simulink model "addFM"  (R2024a)
settings: configuration reference "standardSILConfiguraitonParams" (kept outside this file)
libraries: simulink x2
settings Model: Creator=GTAR  LastModifiedBy=jerem
settings ConfigSetRef: SourceName=standardSILConfiguraitonParams  SourceLocation=Base Workspace

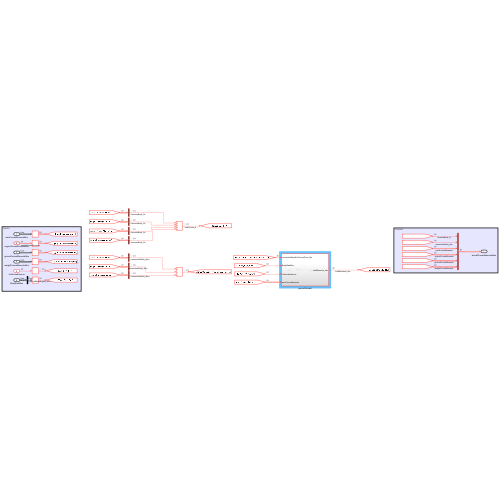
[thumbnail: Simulink's stored preview of the top-level diagram]
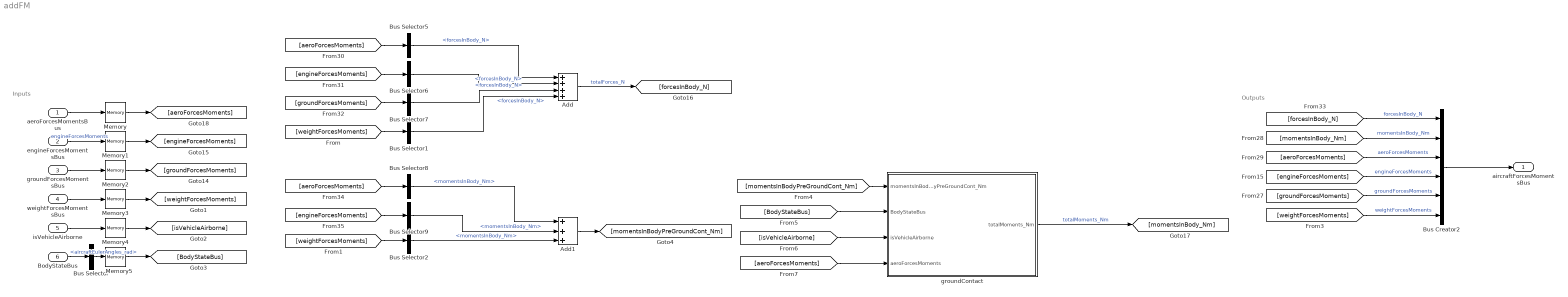
== system addFM ==
  note: Inputs
  note: Outputs
  aeroForcesMomentsBus : Inport  OutDataTypeStr=Bus: ComponentForcesMomentsBus  SampleTime=0
  engineForcesMomentsBus : Inport  Port=2  OutDataTypeStr=Bus: ComponentForcesMomentsBus
  groundForcesMomentsBus : Inport  Port=3  OutDataTypeStr=Bus: ComponentForcesMomentsBus  SampleTime=0
  weightForcesMomentsBus : Inport  Port=4  OutDataTypeStr=Bus: ComponentForcesMomentsBus  SampleTime=0
  isVehicleAirborne : Inport  Port=5  OutDataTypeStr=boolean
  BodyStateBus : Inport  Port=6  OutDataTypeStr=Bus: BodyStateBus  SampleTime=0  BusOutputAsStruct=on
  Add : Sum  Inputs=++++
  Add1 : Sum  Inputs=+++
  Bus Creator2 : BusCreator  Inputs=6  OutDataTypeStr=Bus: AircraftForcesMomentsBus
  Bus Selector : BusSelector  OutputSignals=aircraftEulerAngles_rad
  Bus Selector{1,5..7} (4 alike) : BusSelector  OutputSignals=forcesInBody_N
  Bus Selector2 : BusSelector  OutputSignals=momentsInBody_Nm
  Bus Selector8 : BusSelector  OutputSignals=momentsInBody_Nm
  Bus Selector9 : BusSelector  OutputSignals=momentsInBody_Nm
  Memory{,1..5} (6 alike) : Memory
  groundContact : Subsystem
  aircraftForcesMomentsBus : Outport  OutDataTypeStr=Bus: AircraftForcesMomentsBus  SampleTime=0
  wires:
  [forcesInBody_N] -> Bus Creator2/1  "forcesInBody_N"
  Bus Selector6/1 -> Add/2  "<forcesInBody_N>"
  [engineForcesMoments] -> Bus Creator2/4  "engineForcesMoments"
  [engineForcesMoments] -> Bus Selector9/1
  Bus Selector7/1 -> Add/3  "<forcesInBody_N>"
  [aeroForcesMoments] -> Bus Selector5/1
  Bus Selector9/1 -> Add1/2  "<momentsInBody_Nm>"
  Add/1 -> [forcesInBody_N]  "totalForces_N"
  [aeroForcesMoments] -> Bus Creator2/3  "aeroForcesMoments"
  Bus Selector8/1 -> Add1/1  "<momentsInBody_Nm>"
  [momentsInBody_Nm] -> Bus Creator2/2  "momentsInBody_Nm"
  groundForcesMomentsBus/1 -> Memory2/1
  Bus Creator2/1 -> aircraftForcesMomentsBus/1
  aeroForcesMomentsBus/1 -> Memory/1
  [groundForcesMoments] -> Bus Selector7/1
  engineForcesMomentsBus/1 -> Memory1/1  "engineForcesMoments"
  [aeroForcesMoments] -> Bus Selector8/1
  [engineForcesMoments] -> Bus Selector6/1
  [groundForcesMoments] -> Bus Creator2/5  "groundForcesMoments"
  Memory/1 -> [aeroForcesMoments]
  Memory1/1 -> [engineForcesMoments]
  Memory2/1 -> [groundForcesMoments]
  Memory3/1 -> [weightForcesMoments]
  weightForcesMomentsBus/1 -> Memory3/1
  [weightForcesMoments] -> Bus Selector1/1
  Bus Selector1/1 -> Add/4  "<forcesInBody_N>"
  [weightForcesMoments] -> Bus Selector2/1
  Bus Selector2/1 -> Add1/3  "<momentsInBody_Nm>"
  [weightForcesMoments] -> Bus Creator2/6  "weightForcesMoments"
  Bus Selector5/1 -> Add/1  "<forcesInBody_N>"
  Memory4/1 -> [isVehicleAirborne]
  isVehicleAirborne/1 -> Memory4/1
  groundContact/1(totalMoments_Nm) -> [momentsInBody_Nm]  "totalMoments_Nm"
  Add1/1 -> [momentsInBodyPreGroundCont_Nm]
  BodyStateBus/1 -> Bus Selector/1
  Bus Selector/1 -> Memory5/1  "<aircraftEulerAngles_rad>"
  Memory5/1 -> [BodyStateBus]
  [momentsInBodyPreGroundCont_Nm] -> groundContact/1(momentsInBodyPreGroundCont_Nm)
  [BodyStateBus] -> groundContact/2(BodyStateBus)
  [isVehicleAirborne] -> groundContact/3(isVehicleAirborne)
  [aeroForcesMoments] -> groundContact/4(aeroForcesMoments)

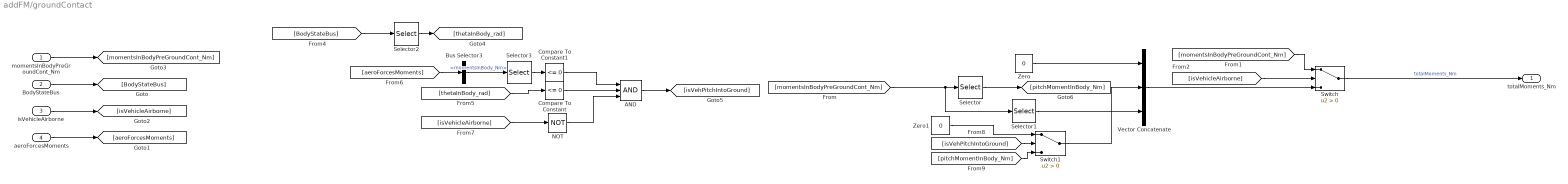
== system addFM/groundContact ==
  momentsInBodyPreGroundCont_Nm : Inport
  BodyStateBus : Inport  Port=2
  isVehicleAirborne : Inport  Port=3
  aeroForcesMoments : Inport  Port=4
  AND : Logic  Inputs=3  AllPortsSameDT=off  OutDataTypeStr=boolean
  Bus Selector3 : BusSelector  OutputSignals=momentsInBody_Nm
  Compare To Constant : simulink/Logic and Bit Operations/Compare To Constant  relop=<=  const=0  OutDataTypeStr=boolean
  Compare To Constant1 : simulink/Logic and Bit Operations/Compare To Constant  relop=<=  const=0  OutDataTypeStr=boolean
  NOT : Logic  Operator=NOT  IconShape=distinctive  AllPortsSameDT=off  OutDataTypeStr=boolean
  Selector : Selector  InputPortWidth=3  IndexOptions=Index vector (dialog)  Indices=2  OutputSizes=1
  Selector1 : Selector  InputPortWidth=3  IndexOptions=Index vector (dialog)  Indices=3  OutputSizes=1
  Selector2 : Selector  InputPortWidth=3  IndexOptions=Index vector (dialog)  Indices=2  OutputSizes=1
  Selector3 : Selector  InputPortWidth=3  IndexOptions=Index vector (dialog)  Indices=2  OutputSizes=1
  Switch : Switch  Criteria=u2 > Threshold  SaturateOnIntegerOverflow=off  InputSameDT=off
  Switch1 : Switch  Criteria=u2 > Threshold  SaturateOnIntegerOverflow=off  InputSameDT=off
  Vector Concatenate : Concatenate  NumInputs=3
  Zero : Constant  Value=0  OutDataTypeStr=Inherit: Inherit via back propagation
  Zero1 : Constant  Value=0  OutDataTypeStr=Inherit: Inherit via back propagation
  totalMoments_Nm : Outport
  wires:
  NOT/1 -> AND/3
  [BodyStateBus] -> Selector2/1
  Compare To Constant/1 -> AND/2
  [thetaInBody_rad] -> Compare To Constant/1
  [isVehicleAirborne] -> NOT/1
  Compare To Constant1/1 -> AND/1
  AND/1 -> [isVehPitchIntoGround]
  [aeroForcesMoments] -> Bus Selector3/1
  Selector3/1 -> Compare To Constant1/1
  Bus Selector3/1 -> Selector3/1  "<momentsInBody_Nm>"
  Selector2/1 -> [thetaInBody_rad]
  [isVehPitchIntoGround] -> Switch1/2
  Zero/1 -> Vector Concatenate/1
  [momentsInBodyPreGroundCont_Nm] -> Selector1/1, Selector/1
  Selector/1 -> [pitchMomentInBody_Nm]
  Switch1/1 -> Vector Concatenate/2
  Selector1/1 -> Vector Concatenate/3
  Zero1/1 -> Switch1/1
  [pitchMomentInBody_Nm] -> Switch1/3
  BodyStateBus/1 -> [BodyStateBus]
  aeroForcesMoments/1 -> [aeroForcesMoments]
  isVehicleAirborne/1 -> [isVehicleAirborne]
  momentsInBodyPreGroundCont_Nm/1 -> [momentsInBodyPreGroundCont_Nm]
  [isVehicleAirborne] -> Switch/2
  Vector Concatenate/1 -> Switch/3
  Switch/1 -> totalMoments_Nm/1  "totalMoments_Nm"
  [momentsInBodyPreGroundCont_Nm] -> Switch/1
